simulink model "suspmodPID"  (Simulink 8.7)
settings: Solver=ode45  SolverMode=SingleTasking  StartTime=0.0  StopTime=50  RelTol=1e-3  AbsTol=1e-6
undefined symbols (not defined in the file): b1, b2, K, k1, k2, m1, m2
settings Model: Creator=Rick  LastModifiedBy=mm395
settings DataIOCC: LimitDataPoints=off  SignalLoggingSaveFormat=ModelDataLogs
settings OptimizationCC: BlockReduction=off  BooleanDataType=off  ExpressionDepthLimit=2147483647
settings DebuggingCC: SaveWithParameterizedLinksMsg=none  SignalResolutionControl=TryResolveAllWithWarning  InheritedTsInSrcMsg=none  MultiTaskDSMMsg=warning  MultiTaskCondExecSysMsg=none  FcnCallInpInsideContextMsg=EnableAllAsWarning  UnknownTsInhSupMsg=none  StateNameClashWarn=warning
settings HardwareCC: TargetUnknown=on

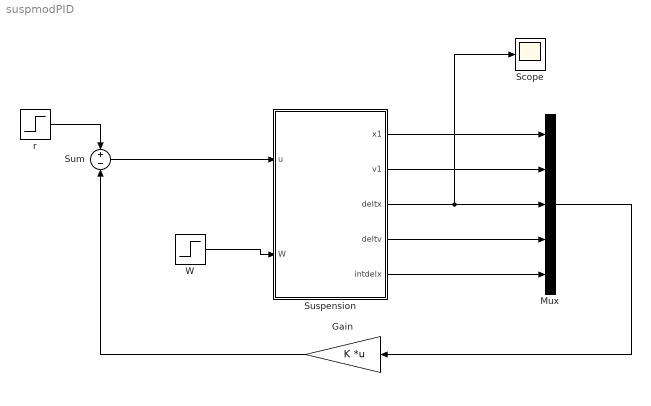
== system suspmodPID ==
  Gain : Gain  Gain=K  Multiplication=Matrix(K*u)
  Mux : Mux  Inputs=5
  Scope : Scope
  Sum : Sum  Inputs=+-
  Suspension : Subsystem
  W : Step  Time=0  After=0.1  SampleTime=0
  r : Step  After=0  SampleTime=0
  wires:
  Suspension/1(x1) -> Mux/1
  Suspension/2(v1) -> Mux/2
  Mux/1 -> Gain/1
  r/1 -> Sum/1
  Gain/1 -> Sum/2
  Sum/1 -> Suspension/1(u)
  W/1 -> Suspension/2(W)
  Suspension/3(deltx) -> Scope/1, Mux/3
  Suspension/4(deltv) -> Mux/4
  Suspension/5(intdelx) -> Mux/5

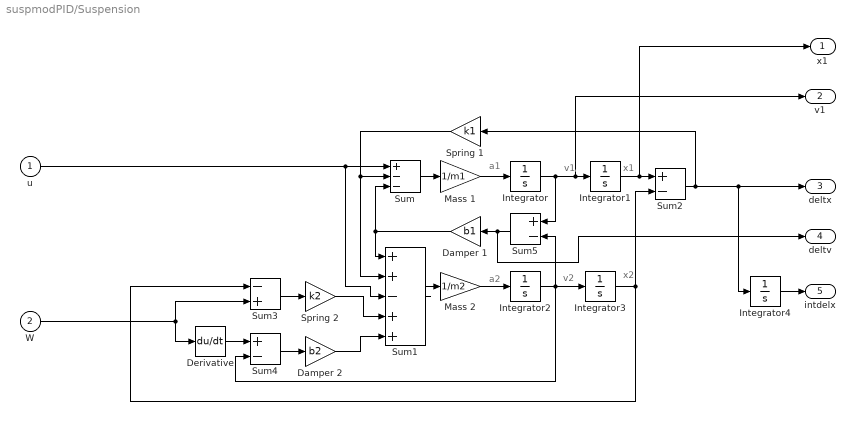
== system suspmodPID/Suspension ==
  note: a1
  note: v1
  note: x1
  note: a2
  note: v2
  note: x2
  u : Inport
  W : Inport  Port=2
  Damper 1 : Gain  Gain=b1  SaturateOnIntegerOverflow=on  OutDataTypeStr=Inherit: Same as input  ParamDataTypeStr=Inherit: Same as input
  Damper 2 : Gain  Gain=b2  SaturateOnIntegerOverflow=on  OutDataTypeStr=Inherit: Same as input  ParamDataTypeStr=Inherit: Same as input
  Derivative : Derivative
  Integrator{,1..4} (5 alike) : Integrator
  Mass 1 : Gain  Gain=1/m1  SaturateOnIntegerOverflow=on  OutDataTypeStr=Inherit: Same as input  ParamDataTypeStr=Inherit: Same as input
  Mass 2 : Gain  Gain=1/m2  SaturateOnIntegerOverflow=on  OutDataTypeStr=Inherit: Same as input  ParamDataTypeStr=Inherit: Same as input
  Spring 1 : Gain  Gain=k1  SaturateOnIntegerOverflow=on  OutDataTypeStr=Inherit: Same as input  ParamDataTypeStr=Inherit: Same as input
  Spring 2 : Gain  Gain=k2  SaturateOnIntegerOverflow=on  OutDataTypeStr=Inherit: Same as input  ParamDataTypeStr=Inherit: Same as input
  Sum : Sum  Inputs=+--  SaturateOnIntegerOverflow=on  InputSameDT=on  OutDataTypeStr=Inherit: Same as first input
  Sum1 : Sum  Inputs=++-++  SaturateOnIntegerOverflow=on  InputSameDT=on  OutDataTypeStr=Inherit: Same as first input
  Sum2 : Sum  Inputs=+-  SaturateOnIntegerOverflow=on  InputSameDT=on  OutDataTypeStr=Inherit: Same as first input
  Sum3 : Sum  Inputs=-+  SaturateOnIntegerOverflow=on  InputSameDT=on  OutDataTypeStr=Inherit: Same as first input
  Sum4 : Sum  Inputs=+-  SaturateOnIntegerOverflow=on  InputSameDT=on  OutDataTypeStr=Inherit: Same as first input
  Sum5 : Sum  Inputs=+-  SaturateOnIntegerOverflow=on  InputSameDT=on  OutDataTypeStr=Inherit: Same as first input
  x1 : Outport  InitialOutput=0
  v1 : Outport  Port=2
  deltx : Outport  Port=3
  deltv : Outport  Port=4
  intdelx : Outport  Port=5
  wires:
  Sum5/1 -> deltv/1, Damper 1/1
  Integrator2/1 -> Integrator3/1, Sum4/2, Sum5/2
  Sum1/1 -> Mass 2/1
  Mass 2/1 -> Integrator2/1
  Damper 1/1 -> Sum1/1, Sum/3
  Mass 1/1 -> Integrator/1
  Sum/1 -> Mass 1/1
  Integrator1/1 -> x1/1, Sum2/1
  Integrator/1 -> v1/1, Integrator1/1, Sum5/1
  Integrator3/1 -> Sum2/2, Sum3/1
  Sum2/1 -> Integrator4/1, deltx/1, Spring 1/1
  Spring 1/1 -> Sum/2, Sum1/2
  Damper 2/1 -> Sum1/5
  Spring 2/1 -> Sum1/4
  Sum3/1 -> Spring 2/1
  Sum4/1 -> Damper 2/1
  u/1 -> Sum/1, Sum1/3
  Derivative/1 -> Sum4/1
  W/1 -> Derivative/1, Sum3/2
  Integrator4/1 -> intdelx/1
